simulink model "sim_double_lin"  (R2015a)
settings: Solver=ode45  StartTime=0.0  StopTime=10  RelTol=1e-10  AbsTol=1e-10
values from neighbouring files (symbols this model uses):
  A = subs(linsys.A0, linvars, WP)    [lin_pendulum.m]    (also in pulley.m = [-D/2, 0; 0, -2/D])
  B = subs(linsys.B0, linvars, WP)    [lin_pendulum.m]
  C = subs(linsys.C0, linvars, WP)    [lin_pendulum.m]    (also in load_lqg.m = dsys.c; run_design.m = disc_ss.c)
  Gamma = dsys.b    [init_values.m]    (also in load_lqg.m; run_design.m = disc_ss.b)
  Ki = -K(:, n+1:end)    [load_control.m]
  Kp = K(:, 1:n)    [load_control.m]
  L = dlqe(Phi, Psi, C, Rw, Rv)    [load_control.m]    (also in load_single_lqg.m = place(dsys.a.', dsys.c.', o_z_poles).'; run_design.m = dlqe(Phi, Psi, alpha*C, Rw, Rv))
  params = params(1:13)    [load_mechanism_params.m]    (also in load_params.m = [g, m0, b0,                m1, I1, b1, L1, L1_cg,           ; load_single_mechanism_params.m = params(1:8); load_single_params.m = [g, m0, b0,                m1, I1, b1, L1, L1_cg,           ; main.m = load_params())
  Phi = dsys.a    [init_values.m]    (also in load_lqg.m; run_design.m = disc_ss.a)
  Psi = [zeros(3, 1); ones(3, 1)]    [load_control.m]    (also in load_lqg.m = [zeros(3); eye(3)]; run_simulink.m = [zeros(3); eye(3)])
  Ts = dsys.ts    [init_values.m]    (also in load_double_sys.m = 0.01; load_lqg.m; load_single_lqg.m; main.m = 0.01)
settings Model: Creator=BPeixoto  LastModifiedBy=brunopeixoto

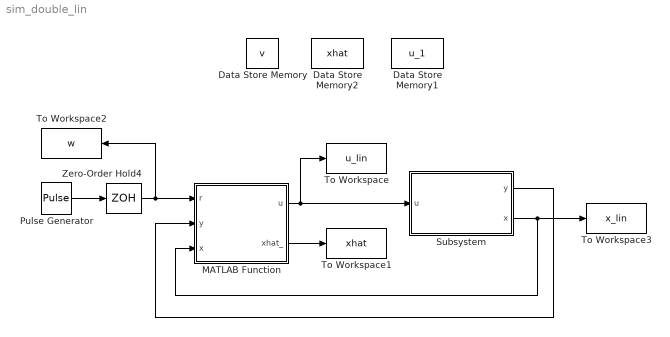
== system sim_double_lin ==
  Data Store Memory : DataStoreMemory  DataStoreName=v  OutDataTypeStr=double
  Data Store Memory1 : DataStoreMemory  DataStoreName=u_1  ReadBeforeWriteMsg=warning  WriteAfterWriteMsg=warning  WriteAfterReadMsg=warning  OutDataTypeStr=double
  Data Store Memory2 : DataStoreMemory  DataStoreName=xhat  ReadBeforeWriteMsg=warning  WriteAfterWriteMsg=warning  WriteAfterReadMsg=warning  InitialValue=params.xhat0  OutDataTypeStr=double
  MATLAB Function : MATLAB Function  TreatAsAtomicUnit=on
  Pulse Generator : DiscretePulseGenerator  PulseType=Time based  Amplitude=params.step_amplitude  Period=10  PulseWidth=50
  Subsystem : Subsystem
  To Workspace : ToWorkspace  VariableName=u_lin  SaveFormat=Structure With Time  SampleTime=-1
  To Workspace1 : ToWorkspace  VariableName=xhat  SaveFormat=Structure With Time  SampleTime=Ts
  To Workspace2 : ToWorkspace  VariableName=w  SaveFormat=Structure With Time  SampleTime=Ts
  To Workspace3 : ToWorkspace  VariableName=x_lin  SaveFormat=Structure With Time  SampleTime=-1
  Zero-Order Hold4 : ZeroOrderHold  SampleTime=Ts
  wires:
  Pulse Generator/1 -> Zero-Order Hold4/1
  Zero-Order Hold4/1 -> MATLAB Function/1(r), To Workspace2/1
  Subsystem/1(y) -> MATLAB Function/2(y)
  MATLAB Function/2(xhat_) -> To Workspace1/1
  MATLAB Function/1(u) -> Subsystem/1(u), To Workspace/1
  Subsystem/2(x) -> To Workspace3/1, MATLAB Function/3(x)

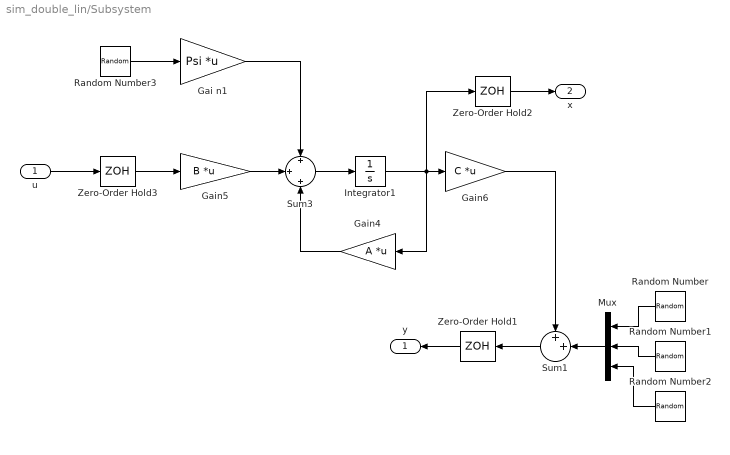
== system sim_double_lin/Subsystem ==
  u : Inport
  Gai n1 : Gain  Gain=Psi  Multiplication=Matrix(K*u) (u vector)
  Gain4 : Gain  Gain=A  Multiplication=Matrix(K*u) (u vector)
  Gain5 : Gain  Gain=B  Multiplication=Matrix(K*u) (u vector)
  Gain6 : Gain  Gain=C  Multiplication=Matrix(K*u) (u vector)
  Integrator1 : Integrator  InitialCondition=params.x0 - [params.q0,params.qp0 ]
  Mux : Mux  Inputs=3
  Random Number : RandomNumber  Variance=params.Rv  SampleTime=Ts
  Random Number1 : RandomNumber  Variance=params.Rv  SampleTime=Ts
  Random Number2 : RandomNumber  Variance=params.Rv  SampleTime=Ts
  Random Number3 : RandomNumber  Variance=params.Rw  SampleTime=Ts
  Sum1 : Sum  Inputs=++|
  Sum3 : Sum  Inputs=+|+|+
  Zero-Order Hold1 : ZeroOrderHold  SampleTime=Ts
  Zero-Order Hold2 : ZeroOrderHold  SampleTime=Ts
  Zero-Order Hold3 : ZeroOrderHold  SampleTime=Ts
  y : Outport
  x : Outport  Port=2
  wires:
  Random Number/1 -> Mux/1
  Gain5/1 -> Sum3/2
  Sum1/1 -> Zero-Order Hold1/1
  Sum3/1 -> Integrator1/1
  Zero-Order Hold3/1 -> Gain5/1
  Mux/1 -> Sum1/2
  Random Number1/1 -> Mux/2
  Gai n1/1 -> Sum3/1
  Random Number2/1 -> Mux/3
  Zero-Order Hold1/1 -> y/1
  Gain4/1 -> Sum3/3
  Random Number3/1 -> Gai n1/1
  u/1 -> Zero-Order Hold3/1
  Zero-Order Hold2/1 -> x/1
  Integrator1/1 -> Zero-Order Hold2/1, Gain4/1, Gain6/1
  Gain6/1 -> Sum1/1

== matlab function sim_double_lin/MATLAB Function ==
  data: r input; u output; xhat_ output; y input; x input; v data_store_memory; Phi parameter; C parameter; L parameter; Gamma parameter; Kp parameter; Ki parameter; xhat data_store_memory
function [u, xhat_] = controle(r, y, x, Phi, C, L, Gamma, Kp, Ki)
    global v xhat;
    
    xhat_ = xhat;
    
%     u = -Kp*x + Ki*v;
    u = -Kp*xhat + Ki*v;

    v = v + r - y(1);
    
    xhat = Phi*xhat + Gamma*u + L*(y - C*xhat);
end
